simulink model "sim_VSS_P"  (R2019a)
settings: Solver=FixedStepAuto  StartTime=0.0  StopTime=50  FixedStep=1e-2  RelTol=1e-3
values from neighbouring files (symbols this model uses):
  a = 47    [mod1s.m]
  b = -35    [mod1s.m]
  C1 = 0.76    [mod1s.m]
  C2 = 11    [mod1s.m]
  h = 4    [mod1s.m]
  K = 19    [mod1s.m]
  T = 29    [mod1s.m]
  x0 = -100    [mod1s.m]
  y0 = 0    [mod1s.m]
  z0 = 0    [mod1s.m]
libraries: simulink_extras x1
settings Model: Creator=ogure  LastModifiedBy=ogure
settings SolverCC: SolverResetMethod=Robust
settings DataIOCC: SaveFormat=Array  SaveOutput=off  ReturnWorkspaceOutputs=off
settings DebuggingCC: SolverPrmCheckMsg=warning

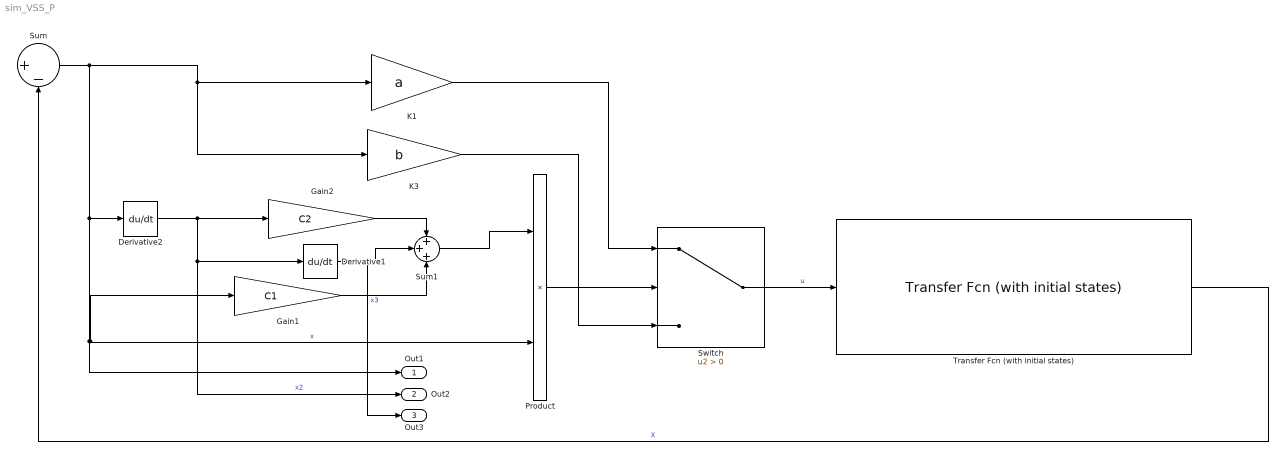
== system sim_VSS_P ==
  Derivative1 : Derivative  CoefficientInTFapproximation=0.00000001
  Derivative2 : Derivative  CoefficientInTFapproximation=0.00000001
  Gain1 : Gain  Gain=C1
  Gain2 : Gain  Gain=C2
  K1 : Gain  Gain=a
  K3 : Gain  Gain=b
  Product : Product
  Sum : Sum  Inputs=|+-
  Sum1 : Sum  Inputs=+++
  Switch : Switch  Criteria=u2 > Threshold  ZeroCross=off
  Transfer Fcn (with initial states) : simulink_extras/Additional Linear/Transfer Fcn (with initial states)  N=[K]  D=[T^2 2*h*T 1 0]  X0=[z0 y0 x0]
  Out1 : Outport  SignalName=X
  Out2 : Outport  Port=2  SignalName=y
  Out3 : Outport  Port=3  SignalName=z
  wires:
  Transfer Fcn (with initial states)/1 -> Sum/2  "X"
  Switch/1 -> Transfer Fcn (with initial states)/1  "u"
  K3/1 -> Switch/3
  Gain2/1 -> Sum1/1
  Derivative2/1 -> Out2/1, Derivative1/1, Gain2/1  "x2"
  Sum1/1 -> Product/1
  Derivative1/1 -> Out3/1, Sum1/2  "x3"
  Product/1 -> Switch/2
  Gain1/1 -> Sum1/3
  Sum/1 -> Out1/1, Gain1/1, Product/2, Derivative2/1, K3/1, K1/1  "x"
  K1/1 -> Switch/1
